simulink model "attitude_controller"  (R2015a)
settings: Solver=ode45  StartTime=0.0  StopTime=10.0  RelTol=1e-3
values from neighbouring files (symbols this model uses):
  AC_ATTITUDE_ACCEL_RP_CONTROLLER_MAX_RADSS = 720    [arducopter_initialization.m]    (also in startup.m)
  AC_ATTITUDE_ACCEL_RP_CONTROLLER_MIN_RADDS = 40    [arducopter_initialization.m]    (also in startup.m)
  AC_ATTITUDE_ACCEL_Y_CONTROLLER_MAX_RADSS = 120    [arducopter_initialization.m]    (also in startup.m)
  AC_ATTITUDE_ACCEL_Y_CONTROLLER_MIN_RADSS = 10    [arducopter_initialization.m]    (also in startup.m)
  ATC_ACCEL_P_MAX = 72000    [arducopter_initialization.m]    (also in startup.m)
  ATC_ACCEL_R_MAX = 72000    [arducopter_initialization.m]    (also in startup.m)
  ATC_ACCEL_Y_MAX = 36000    [arducopter_initialization.m]    (also in startup.m)
  ATC_ANG_PIT_P = 4.5000    (= 4.5)    [arducopter_initialization.m]    (also in startup.m)
  ATC_ANG_RLL_P = 4.5000    (= 4.5)    [arducopter_initialization.m]    (also in startup.m)
  ATC_ANG_YAW_P = 4.5000    (= 4.5)    [arducopter_initialization.m]    (also in startup.m)
  dt = 0.01    [arducopter_initialization.m]    (also in startup.m)
  p_angle_yaw_kp = 0.01    [arducopter_initialization.m]
  smoothing_gain = 1    [arducopter_initialization.m]    (also in startup.m)
undefined symbols (not defined in the file or in its folder): AC_ATTITUDE_THRUST_ERROR_ANGLE
libraries: arducopter_library x21, simulink x5, simulink_extras x4
settings Model: Creator=anne  LastModifiedBy=pa872d
settings DataIOCC: LimitDataPoints=off  SaveFormat=Dataset
settings HardwareCC: ProdBitPerPointer=64  ProdLargestAtomicFloat=Float  ProdIntDivRoundTo=Zero  ProdEndianess=LittleEndian  ProdHWDeviceType=Specified
settings ModelReferenceCC: PropagateSignalLabelsOutOfModel=on
settings GRTTargetCC: GeneratePreprocessorConditionals=Use local settings

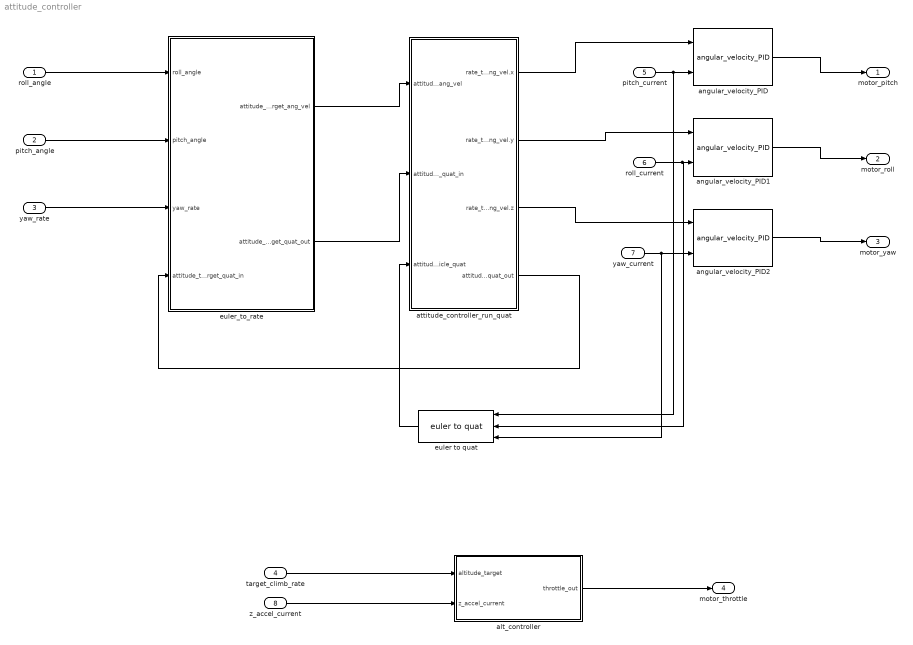
== system attitude_controller ==
  roll_angle : Inport
  pitch_angle : Inport  Port=2
  yaw_rate : Inport  Port=3
  target_climb_rate : Inport  Port=4
  pitch_current : Inport  Port=5
  roll_current : Inport  Port=6
  yaw_current : Inport  Port=7
  z_accel_current : Inport  Port=8
  alt_controller : Subsystem
  angular_velocity_PID : arducopter_library/angular_velocity_PID  P_rate=0  I_rate=0  D_rate=0  N=0
  angular_velocity_PID1 : arducopter_library/angular_velocity_PID  P_rate=0  I_rate=0  D_rate=0  N=0
  angular_velocity_PID2 : arducopter_library/angular_velocity_PID  P_rate=0  I_rate=0  D_rate=0  N=0
  attitude_controller_run_quat : Subsystem
  euler to quat : arducopter_library/euler to quat  SystemSampleTime=-1
  euler_to_rate : Subsystem  Variant=on
  motor_pitch : Outport
  motor_roll : Outport  Port=2
  motor_yaw : Outport  Port=3
  motor_throttle : Outport  Port=4
  wires:
  target_climb_rate/1 -> alt_controller/1(altitude_target)
  roll_angle/1 -> euler_to_rate/1(roll_angle)
  pitch_angle/1 -> euler_to_rate/2(pitch_angle)
  yaw_rate/1 -> euler_to_rate/3(yaw_rate)
  alt_controller/1(throttle_out) -> motor_throttle/1
  angular_velocity_PID2/1 -> motor_yaw/1
  angular_velocity_PID/1 -> motor_pitch/1
  angular_velocity_PID1/1 -> motor_roll/1
  yaw_current/1 -> euler to quat/3, angular_velocity_PID2/2
  pitch_current/1 -> euler to quat/1, angular_velocity_PID/2
  roll_current/1 -> euler to quat/2, angular_velocity_PID1/2
  z_accel_current/1 -> alt_controller/2(z_accel_current)
  attitude_controller_run_quat/1(rate_target_ang_vel.x) -> angular_velocity_PID/1
  attitude_controller_run_quat/2(rate_target_ang_vel.y) -> angular_velocity_PID1/1
  attitude_controller_run_quat/3(rate_target_ang_vel.z) -> angular_velocity_PID2/1
  attitude_controller_run_quat/4(attitude_target_quat_out) -> euler_to_rate/4(attitude_target_quat_in)
  euler_to_rate/2(attitude_target_quat_out) -> attitude_controller_run_quat/2(attitude_target_quat_in)
  euler_to_rate/1(attitude_target_ang_vel) -> attitude_controller_run_quat/1(attitude_target_ang_vel)
  euler to quat/1 -> attitude_controller_run_quat/3(attitude_vehicle_quat)

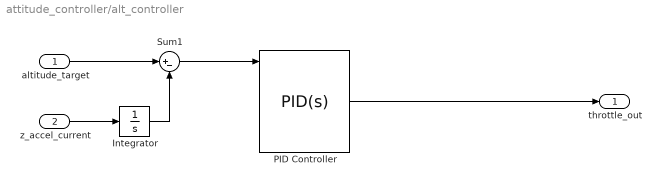
== system attitude_controller/alt_controller ==
  altitude_target : Inport
  z_accel_current : Inport  Port=2
  Integrator : Integrator
  PID Controller : simulink/Continuous/PID Controller  Controller=PID  TimeDomain=Continuous-time  SampleTime=-1  IntegratorMethod=Forward Euler  FilterMethod=Forward Euler  Form=Parallel  UseFilter=on  ControllerParametersSource=external  P=1  I=1  D=0  N=100  InitialConditionSource=internal  InitialConditionForIntegrator=0  InitialConditionForFilter=0  ExternalReset=none  LimitOutput=off  UpperSaturationLimit=inf  LowerSaturationLimit=-inf  LinearizeAsGain=on  AntiWindupMode=none  Kb=1  TrackingMode=off  Kt=1  PParamMin=[]  PParamMax=[]  IParamMin=[]  IParamMax=[]  DParamMin=[]  DParamMax=[]  NParamMin=[]  NParamMax=[]  KbParamMin=[]  KbParamMax=[]  KtParamMin=[]  KtParamMax=[]  POutMin=[]  POutMax=[]  IOutMin=[]  IOutMax=[]  DOutMin=[]  DOutMax=[]  NOutMin=[]  NOutMax=[]  KbOutMin=[]  KbOutMax=[]  KtOutMin=[]  KtOutMax=[]  IntegratorOutMin=[]  IntegratorOutMax=[]  FilterOutMin=[]  FilterOutMax=[]  SumOutMin=[]  SumOutMax=[]  SumI1OutMin=[]  SumI1OutMax=[]  SumI2OutMin=[]  SumI2OutMax=[]  SumI3OutMin=[]  SumI3OutMax=[]  SumDOutMin=[]  SumDOutMax=[]  SaturationOutMin=[]  SaturationOutMax=[]  IntegratorContinuousStateAttributes=''  IntegratorStateMustResolveToSignalObject=off  IntegratorRTWStateStorageClass=Auto  FilterContinuousStateAttributes=''  FilterStateMustResolveToSignalObject=off  FilterRTWStateStorageClass=Auto  DifferentiatorICPrevScaledInput=0  DifferentiatorOutMin=[]  DifferentiatorOutMax=[]
  Sum1 : Sum  Inputs=|+-
  throttle_out : Outport
  wires:
  PID Controller/1 -> throttle_out/1
  altitude_target/1 -> Sum1/1
  Sum1/1 -> PID Controller/1
  z_accel_current/1 -> Integrator/1
  Integrator/1 -> Sum1/2

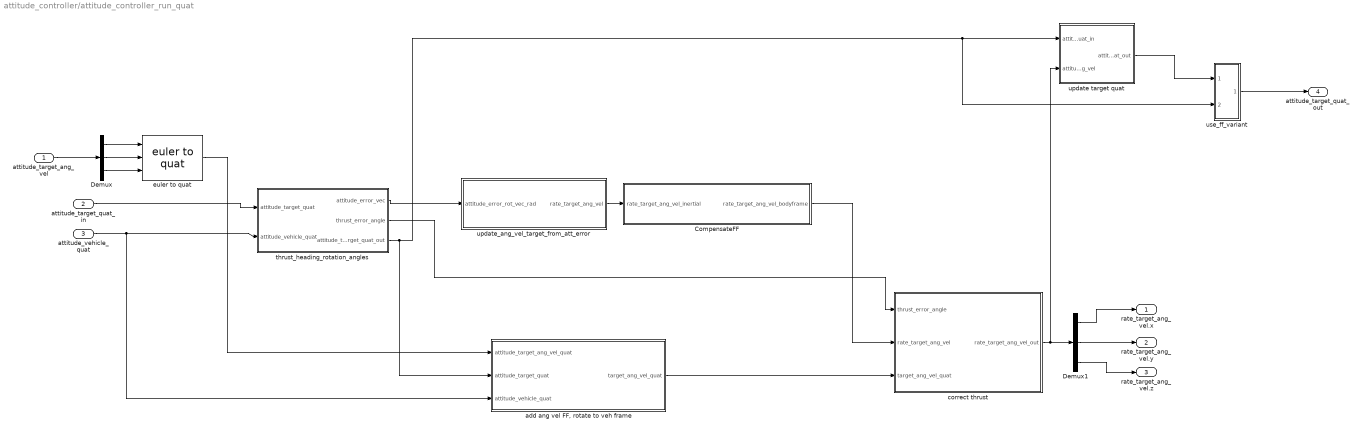
== system attitude_controller/attitude_controller_run_quat ==
  attitude_target_ang_vel : Inport
  attitude_target_quat_in : Inport  Port=2
  attitude_vehicle_quat : Inport  Port=3
  CompensateFF : Subsystem
  Demux : Demux  Outputs=3
  Demux1 : Demux  Outputs=3
  "add ang vel FF, rotate to veh frame" : MATLAB Function  TreatAsAtomicUnit=on
      settings: PermitHierarchicalResolution=ParametersOnly
  correct thrust : Subsystem
  euler to quat : arducopter_library/euler to quat  SystemSampleTime=-1
  thrust_heading_rotation_angles : Subsystem
  update target quat : Subsystem
  update_ang_vel_target_from_att_error : Subsystem  Variant=on
  use_ff_variant : Subsystem  Description=Replaced Block  mask(Replaced Block){}
      mask help: This block has been replaced with an empty subsystem because it used functionality that is unavailable in Simulink R2015a.
      mask Display: fprintf('Replaced: %s\n','VariantSource')
  rate_target_ang_vel.x : Outport
  rate_target_ang_vel.y : Outport  Port=2
  rate_target_ang_vel.z : Outport  Port=3
  attitude_target_quat_out : Outport  Port=4
  wires:
  attitude_target_ang_vel/1 -> Demux/1
  attitude_vehicle_quat/1 -> "add ang vel FF, rotate to veh frame"/3(attitude_vehicle_quat), thrust_heading_rotation_angles/2(attitude_vehicle_quat)
  attitude_target_quat_in/1 -> thrust_heading_rotation_angles/1(attitude_target_quat)
  thrust_heading_rotation_angles/1(attitude_error_vec) -> update_ang_vel_target_from_att_error/1(attitude_error_rot_vec_rad)
  Demux/1 -> euler to quat/1
  Demux/2 -> euler to quat/2
  Demux/3 -> euler to quat/3
  euler to quat/1 -> "add ang vel FF, rotate to veh frame"/1(attitude_target_ang_vel_quat)
  update_ang_vel_target_from_att_error/1(rate_target_ang_vel) -> CompensateFF/1(rate_target_ang_vel_inertial)
  "add ang vel FF, rotate to veh frame"/1(target_ang_vel_quat) -> correct thrust/3(target_ang_vel_quat)
  CompensateFF/1(rate_target_ang_vel_bodyframe) -> correct thrust/2(rate_target_ang_vel)
  thrust_heading_rotation_angles/2(thrust_error_angle) -> correct thrust/1(thrust_error_angle)
  correct thrust/1(rate_target_ang_vel_out) -> update target quat/2(attitude_target_ang_vel), Demux1/1
  Demux1/1 -> rate_target_ang_vel.x/1
  Demux1/2 -> rate_target_ang_vel.y/1
  Demux1/3 -> rate_target_ang_vel.z/1
  use_ff_variant/1(Out1) -> attitude_target_quat_out/1
  update target quat/1(attitude_target_quat_out) -> use_ff_variant/1(In1)
  thrust_heading_rotation_angles/3(attitude_target_quat_out) -> "add ang vel FF, rotate to veh frame"/2(attitude_target_quat), use_ff_variant/2(In2), update target quat/1(attitude_target_quat_in)

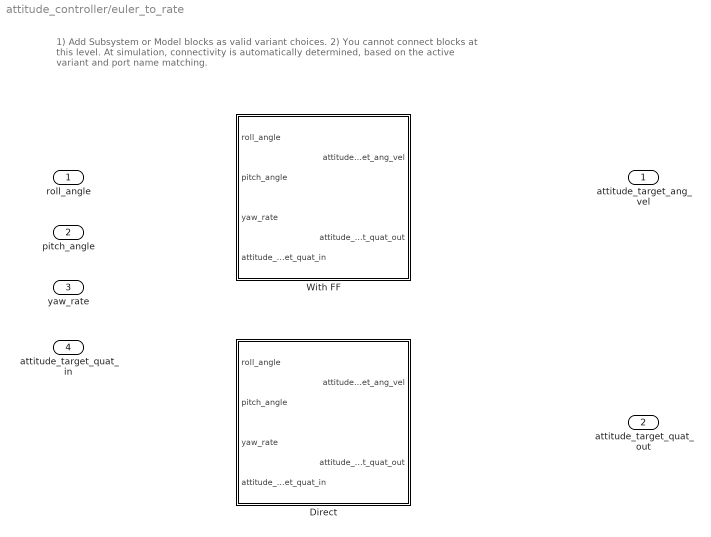
== system attitude_controller/euler_to_rate ==
  note: 1) Add Subsystem or Model blocks as valid variant choices.
      | 2) You cannot connect blocks at this level. At simulation, connectivity is automatically
      | determined, based on the active variant and port name matching.
  roll_angle : Inport
  pitch_angle : Inport  Port=2
  yaw_rate : Inport  Port=3
  attitude_target_quat_in : Inport  Port=4
  Direct : Subsystem  VariantControl=USE_DIRECT_VARIANT
  With FF : Subsystem  VariantControl=USE_FF_VARIANT
  attitude_target_ang_vel : Outport
  attitude_target_quat_out : Outport  Port=2

== system attitude_controller/attitude_controller_run_quat/CompensateFF ==
  note: This function should add a feed forward term that ensures the roll and pitch errors rotate with the body fram instead of the reference frame
  rate_target_ang_vel_inertial : Inport
  rate_target_ang_vel_bodyframe : Outport
  wires:
  rate_target_ang_vel_inertial/1 -> rate_target_ang_vel_bodyframe/1

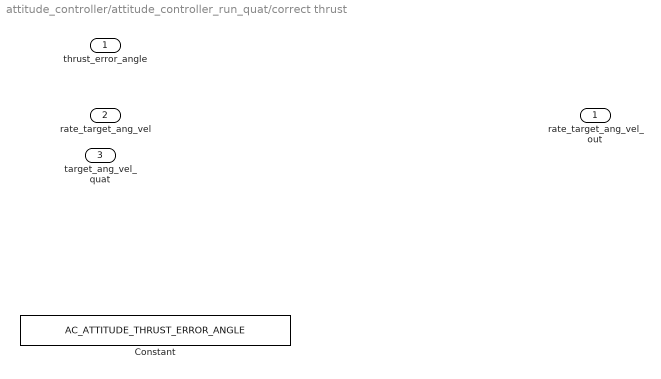
== system attitude_controller/attitude_controller_run_quat/correct thrust ==
  thrust_error_angle : Inport
  rate_target_ang_vel : Inport  Port=2
  target_ang_vel_quat : Inport  Port=3
  Constant : Constant  Value=AC_ATTITUDE_THRUST_ERROR_ANGLE
  rate_target_ang_vel_out : Outport

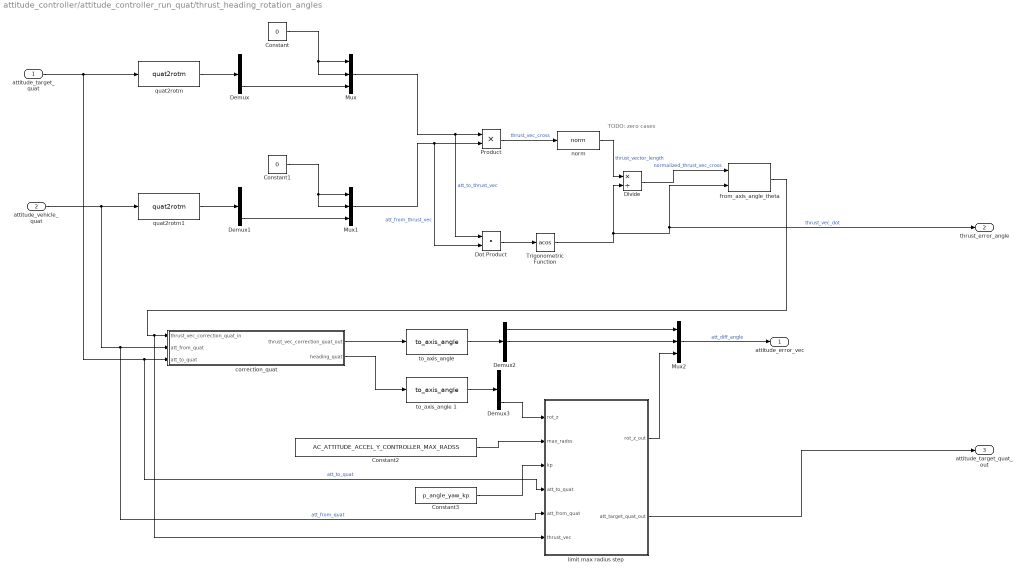
== system attitude_controller/attitude_controller_run_quat/thrust_heading_rotation_angles ==
  note: TODO: zero cases
  attitude_target_quat : Inport
  attitude_vehicle_quat : Inport  Port=2
  Constant : Constant  Value=0
  Constant1 : Constant  Value=0
  Constant2 : Constant  Value=AC_ATTITUDE_ACCEL_Y_CONTROLLER_MAX_RADSS
  Constant3 : Constant  Value=p_angle_yaw_kp
  Demux{,1..3} (4 alike) : Demux  Outputs=3
  Divide : Product  Inputs=*/
  Dot Product : DotProduct  OutMin=-1  OutMax=1  InputSameDT=on  OutDataTypeStr=Inherit: Inherit via internal rule
  Mux : Mux  Inputs=3
  Mux1 : Mux  Inputs=3
  Mux2 : Mux  Inputs=3
  Product : Product
  Trigonometric Function : Trigonometry  Operator=acos
  correction_quat : MATLAB Function  TreatAsAtomicUnit=on
      settings: PermitHierarchicalResolution=ParametersOnly
  from_axis_angle_theta : arducopter_library/from_axis_angle_theta
  limit max radius step : MATLAB Function  TreatAsAtomicUnit=on
      settings: PermitHierarchicalResolution=ParametersOnly
  "norm " : MATLABFcn  MATLABFcn=norm
  quat2rotm : arducopter_library/quat2rotm  SystemSampleTime=-1
  quat2rotm1 : arducopter_library/quat2rotm  SystemSampleTime=-1
  "to_axis_angle " : arducopter_library/to_axis_angle 
  to_axis_angle 1 : arducopter_library/to_axis_angle 
  attitude_error_vec : Outport
  thrust_error_angle : Outport  Port=2
  attitude_target_quat_out : Outport  Port=3
  wires:
  attitude_target_quat/1 -> limit max radius step/4(att_to_quat), correction_quat/3(att_to_quat), quat2rotm/1  "att_to_quat"
  attitude_vehicle_quat/1 -> limit max radius step/5(att_from_quat), correction_quat/2(att_from_quat), quat2rotm1/1  "att_from_quat"
  Mux2/1 -> attitude_error_vec/1  "att_diff_angle"
  Trigonometric Function/1 -> from_axis_angle_theta/2, thrust_error_angle/1, Divide/2  "thrust_vec_dot"
  quat2rotm/1 -> Demux/1
  Demux/3 -> Mux/3
  Constant/1 -> Mux/2, Mux/1
  Mux/1 -> Dot Product/1, Product/1  "att_to_thrust_vec"
  quat2rotm1/1 -> Demux1/1
  Demux1/3 -> Mux1/3
  Constant1/1 -> Mux1/2, Mux1/1
  Mux1/1 -> Dot Product/2, Product/2  "att_from_thrust_vec"
  Product/1 -> "norm "/1  "thrust_vec_cross"
  Dot Product/1 -> Trigonometric Function/1
  "norm "/1 -> Divide/1  "thrust_vector_length"
  Divide/1 -> from_axis_angle_theta/1  "normalized_thrust_vec_cross"
  from_axis_angle_theta/1 -> limit max radius step/6(thrust_vec), correction_quat/1(thrust_vec_correction_quat_in)
  correction_quat/1(thrust_vec_correction_quat_out) -> "to_axis_angle "/1
  "to_axis_angle "/1 -> Demux2/1
  Demux2/1 -> Mux2/1
  Demux2/2 -> Mux2/2
  correction_quat/2(heading_quat) -> to_axis_angle 1/1
  to_axis_angle 1/1 -> Demux3/1
  Demux3/3 -> limit max radius step/1(rot_z)
  Constant2/1 -> limit max radius step/2(max_radss)
  Constant3/1 -> limit max radius step/3(kp)
  limit max radius step/1(rot_z_out) -> Mux2/3
  limit max radius step/2(att_target_quat_out) -> attitude_target_quat_out/1

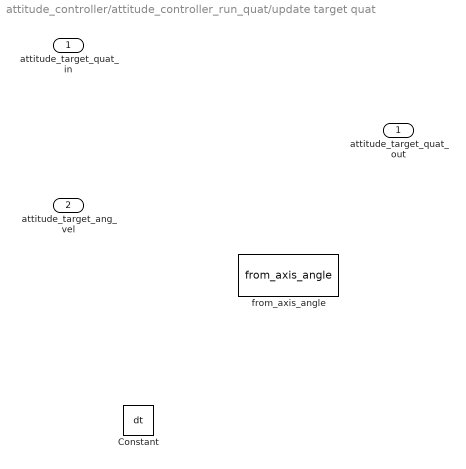
== system attitude_controller/attitude_controller_run_quat/update target quat ==
  attitude_target_quat_in : Inport
  attitude_target_ang_vel : Inport  Port=2
  Constant : Constant  Value=dt
  from_axis_angle : arducopter_library/from_axis_angle  SystemSampleTime=-1
  attitude_target_quat_out : Outport

== system attitude_controller/attitude_controller_run_quat/update_ang_vel_target_from_att_error ==
  note: 1) Add Subsystem or Model blocks as valid variant choices.
      | 2) You cannot connect blocks at this level. At simulation, connectivity is automatically
      | determined, based on the active variant and port name matching.
  attitude_error_rot_vec_rad : Inport
  shaped : Subsystem  VariantControl=USE_FF_VARIANT
  unshaped : Subsystem  VariantControl=USE_DIRECT_VARIANT
  rate_target_ang_vel : Outport

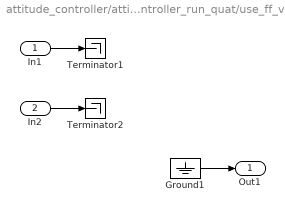
== system attitude_controller/attitude_controller_run_quat/use_ff_variant ==
  In1 : Inport
  In2 : Inport  Port=2
  Ground1 : Ground
  Terminator1 : Terminator
  Terminator2 : Terminator
  Out1 : Outport
  wires:
  Ground1/1 -> Out1/1
  In2/1 -> Terminator2/1
  In1/1 -> Terminator1/1

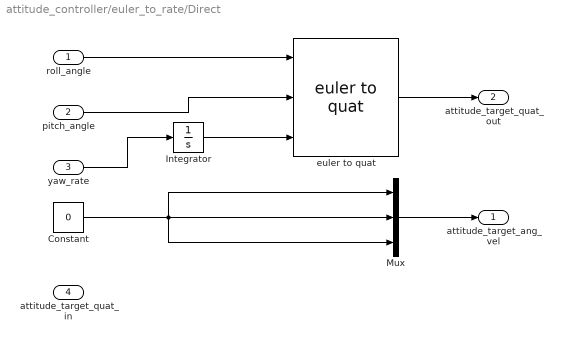
== system attitude_controller/euler_to_rate/Direct ==
  roll_angle : Inport
  pitch_angle : Inport  Port=2
  yaw_rate : Inport  Port=3
  attitude_target_quat_in : Inport  Port=4
  Constant : Constant  Value=0
  Integrator : Integrator
  Mux : Mux  Inputs=3
  euler to quat : arducopter_library/euler to quat  SystemSampleTime=-1
  attitude_target_ang_vel : Outport
  attitude_target_quat_out : Outport  Port=2
  wires:
  roll_angle/1 -> euler to quat/1
  pitch_angle/1 -> euler to quat/2
  Constant/1 -> Mux/3, Mux/2, Mux/1
  Integrator/1 -> euler to quat/3
  yaw_rate/1 -> Integrator/1
  euler to quat/1 -> attitude_target_quat_out/1
  Mux/1 -> attitude_target_ang_vel/1

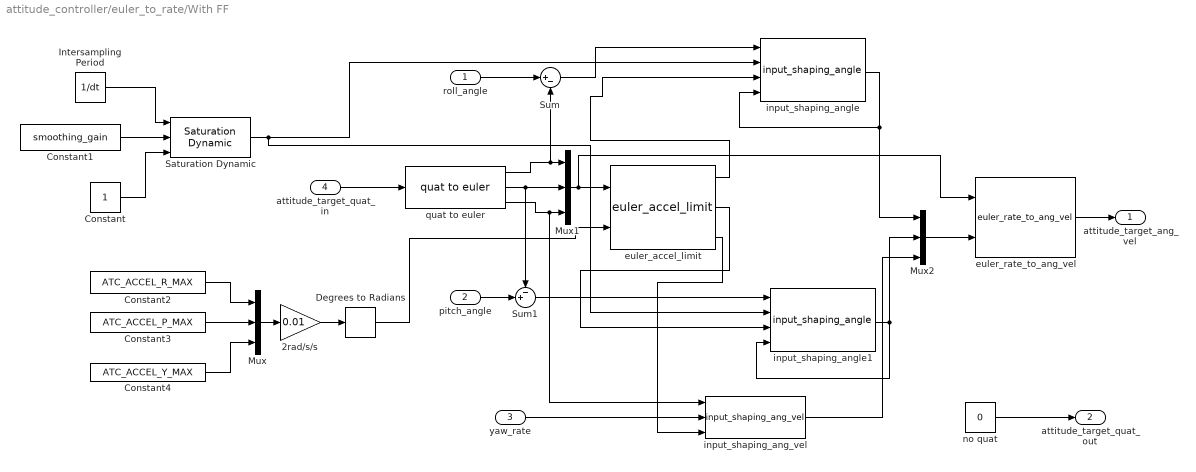
== system attitude_controller/euler_to_rate/With FF ==
  roll_angle : Inport
  pitch_angle : Inport  Port=2
  yaw_rate : Inport  Port=3
  attitude_target_quat_in : Inport  Port=4
  2rad/s/s : Gain  Gain=0.01
  Constant : Constant
  Constant1 : Constant  Value=smoothing_gain
  Constant2 : Constant  Value=ATC_ACCEL_R_MAX
  Constant3 : Constant  Value=ATC_ACCEL_P_MAX
  Constant4 : Constant  Value=ATC_ACCEL_Y_MAX
  Degrees to Radians : simulink_extras/Transformations/Degrees to Radians
  Intersampling Period : Constant  Value=1/dt
  Mux : Mux  Inputs=3
  Mux1 : Mux  Inputs=3
  Mux2 : Mux  Inputs=3
  Saturation Dynamic : simulink/Discontinuities/Saturation Dynamic  OutMin=[]  OutMax=[]  OutDataTypeStr=Inherit: Same as second input  OutDataType=fixdt(1, 16)  OutScaling=2^-10  DoSatur=off
  Sum : Sum  Inputs=|+-
  Sum1 : Sum  Inputs=-+|
  euler_accel_limit : arducopter_library/euler_accel_limit  SystemSampleTime=-1
  euler_rate_to_ang_vel : arducopter_library/euler_rate_to_ang_vel  SystemSampleTime=-1
  input_shaping_ang_vel : arducopter_library/input_shaping_ang_vel  SystemSampleTime=-1
  input_shaping_angle : arducopter_library/input_shaping_angle  SystemSampleTime=-1
  input_shaping_angle1 : arducopter_library/input_shaping_angle  SystemSampleTime=-1
  no quat : Constant  Value=0
  quat to euler : arducopter_library/quat to euler  SystemSampleTime=-1
  attitude_target_ang_vel : Outport
  attitude_target_quat_out : Outport  Port=2
  wires:
  Constant1/1 -> Saturation Dynamic/2
  attitude_target_quat_in/1 -> quat to euler/1
  Constant/1 -> Saturation Dynamic/3
  Intersampling Period/1 -> Saturation Dynamic/1
  roll_angle/1 -> Sum/1
  pitch_angle/1 -> Sum1/2
  yaw_rate/1 -> input_shaping_ang_vel/2
  quat to euler/1 -> Sum/2, Mux1/1
  quat to euler/2 -> Sum1/1, Mux1/2
  quat to euler/3 -> input_shaping_ang_vel/1, Mux1/3
  Mux1/1 -> euler_rate_to_ang_vel/1, euler_accel_limit/1
  Sum/1 -> input_shaping_angle/1
  Saturation Dynamic/1 -> input_shaping_angle1/2, input_shaping_angle/2
  euler_accel_limit/1 -> input_shaping_angle/3
  input_shaping_angle/1 -> Mux2/1, input_shaping_angle/4
  Sum1/1 -> input_shaping_angle1/1
  euler_accel_limit/2 -> input_shaping_angle1/3
  input_shaping_angle1/1 -> input_shaping_angle1/4, Mux2/2
  euler_accel_limit/3 -> input_shaping_ang_vel/3
  input_shaping_ang_vel/1 -> Mux2/3
  Mux2/1 -> euler_rate_to_ang_vel/2
  euler_rate_to_ang_vel/1 -> attitude_target_ang_vel/1
  no quat/1 -> attitude_target_quat_out/1
  Mux/1 -> 2rad/s/s/1
  Constant2/1 -> Mux/1
  Constant3/1 -> Mux/2
  Constant4/1 -> Mux/3
  2rad/s/s/1 -> Degrees to Radians/1
  Degrees to Radians/1 -> euler_accel_limit/2

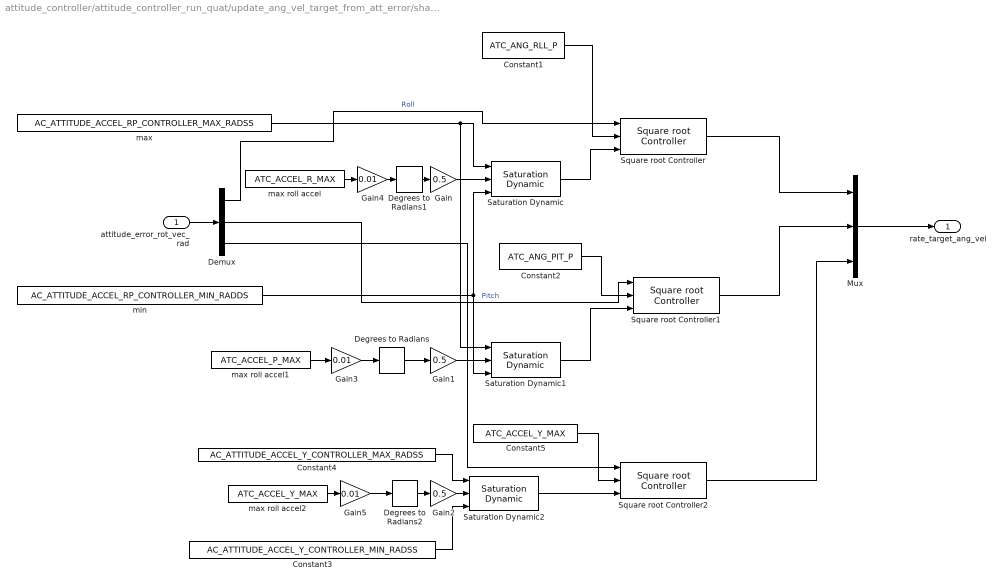
== system attitude_controller/attitude_controller_run_quat/update_ang_vel_target_from_att_error/shaped ==
  attitude_error_rot_vec_rad : Inport
  Constant1 : Constant  Value=ATC_ANG_RLL_P
  Constant2 : Constant  Value=ATC_ANG_PIT_P
  Constant3 : Constant  Value=AC_ATTITUDE_ACCEL_Y_CONTROLLER_MIN_RADSS
  Constant4 : Constant  Value=AC_ATTITUDE_ACCEL_Y_CONTROLLER_MAX_RADSS
  Constant5 : Constant  Value=ATC_ACCEL_Y_MAX
  Degrees to Radians : simulink_extras/Transformations/Degrees to Radians
  Degrees to Radians1 : simulink_extras/Transformations/Degrees to Radians
  Degrees to Radians2 : simulink_extras/Transformations/Degrees to Radians
  Demux : Demux  Outputs=3
  Gain : Gain  Gain=0.5
  Gain1 : Gain  Gain=0.5
  Gain2 : Gain  Gain=0.5
  Gain3 : Gain  Gain=0.01
  Gain4 : Gain  Gain=0.01
  Gain5 : Gain  Gain=0.01
  Mux : Mux  Inputs=3
  Saturation Dynamic : simulink/Discontinuities/Saturation Dynamic  OutMin=[]  OutMax=[]  OutDataTypeStr=Inherit: Same as second input  OutDataType=fixdt(1, 16)  OutScaling=2^-10  DoSatur=off
  Saturation Dynamic1 : simulink/Discontinuities/Saturation Dynamic  OutMin=[]  OutMax=[]  OutDataTypeStr=Inherit: Same as second input  OutDataType=fixdt(1, 16)  OutScaling=2^-10  DoSatur=off
  Saturation Dynamic2 : simulink/Discontinuities/Saturation Dynamic  OutMin=[]  OutMax=[]  OutDataTypeStr=Inherit: Same as second input  OutDataType=fixdt(1, 16)  OutScaling=2^-10  DoSatur=off
  Square root Controller : arducopter_library/Square root Controller  SystemSampleTime=-1
  Square root Controller1 : arducopter_library/Square root Controller  SystemSampleTime=-1
  Square root Controller2 : arducopter_library/Square root Controller  SystemSampleTime=-1
  max : Constant  Value=AC_ATTITUDE_ACCEL_RP_CONTROLLER_MAX_RADSS
  max roll accel : Constant  Value=ATC_ACCEL_R_MAX
  max roll accel1 : Constant  Value=ATC_ACCEL_P_MAX
  max roll accel2 : Constant  Value=ATC_ACCEL_Y_MAX
  min : Constant  Value=AC_ATTITUDE_ACCEL_RP_CONTROLLER_MIN_RADDS
  rate_target_ang_vel : Outport
  wires:
  attitude_error_rot_vec_rad/1 -> Demux/1
  Saturation Dynamic/1 -> Square root Controller/3
  Gain/1 -> Saturation Dynamic/2
  max/1 -> Saturation Dynamic1/1, Saturation Dynamic/1
  min/1 -> Saturation Dynamic/3, Saturation Dynamic1/3
  Demux/1 -> Square root Controller/1  "Roll"
  Saturation Dynamic1/1 -> Square root Controller1/3
  Gain1/1 -> Saturation Dynamic1/2
  Demux/2 -> Square root Controller1/1  "Pitch"
  Constant1/1 -> Square root Controller/2
  Constant2/1 -> Square root Controller1/2
  Saturation Dynamic2/1 -> Square root Controller2/3
  Gain2/1 -> Saturation Dynamic2/2
  Constant4/1 -> Saturation Dynamic2/1
  Constant3/1 -> Saturation Dynamic2/3
  Demux/3 -> Square root Controller2/1
  Constant5/1 -> Square root Controller2/2
  Mux/1 -> rate_target_ang_vel/1
  Square root Controller/1 -> Mux/1
  Square root Controller1/1 -> Mux/2
  Square root Controller2/1 -> Mux/3
  Gain3/1 -> Degrees to Radians/1
  max roll accel1/1 -> Gain3/1
  Degrees to Radians/1 -> Gain1/1
  Gain4/1 -> Degrees to Radians1/1
  max roll accel/1 -> Gain4/1
  Degrees to Radians1/1 -> Gain/1
  Gain5/1 -> Degrees to Radians2/1
  Degrees to Radians2/1 -> Gain2/1
  max roll accel2/1 -> Gain5/1

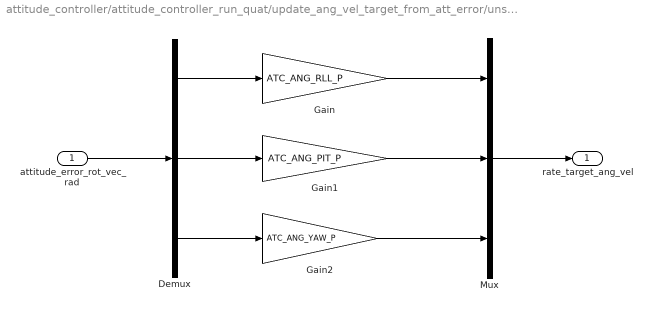
== system attitude_controller/attitude_controller_run_quat/update_ang_vel_target_from_att_error/unshaped ==
  attitude_error_rot_vec_rad : Inport
  Demux : Demux  Outputs=3
  Gain : Gain  Gain=ATC_ANG_RLL_P
  Gain1 : Gain  Gain=ATC_ANG_PIT_P
  Gain2 : Gain  Gain=ATC_ANG_YAW_P
  Mux : Mux  Inputs=3
  rate_target_ang_vel : Outport
  wires:
  attitude_error_rot_vec_rad/1 -> Demux/1
  Demux/1 -> Gain/1
  Gain/1 -> Mux/1
  Demux/2 -> Gain1/1
  Demux/3 -> Gain2/1
  Gain2/1 -> Mux/3
  Gain1/1 -> Mux/2
  Mux/1 -> rate_target_ang_vel/1

== matlab function attitude_controller/attitude_controller_run_quat/thrust_heading_rotation_angles/correction_quat ==
  data: thrust_vec_correction_quat_in input; thrust_vec_correction_quat_out output; att_from_quat input; heading_quat output; att_to_quat input
function [thrust_vec_correction_quat_out, heading_quat] = fcn(thrust_vec_correction_quat_in, att_from_quat, att_to_quat)
thrust_vec_correction_quat_out = att_from_quat \ thrust_vec_correction_quat_in * att_from_quat;

% calculate the remaining rotation required after thrust vector is rotated
heading_quat = thrust_vec_correction_quat_out \ att_from_quat \ att_to_quat;

== matlab function attitude_controller/attitude_controller_run_quat/add ang vel FF, rotate to veh frame ==
  data: attitude_target_ang_vel_quat input; attitude_target_quat input; target_ang_vel_quat output; attitude_vehicle_quat input
function target_ang_vel_quat = fcn(attitude_target_ang_vel_quat,...
                                attitude_target_quat, ...
                                attitude_vehicle_quat)


attitude_error_quat = inverse(attitude_vehicle_quat) * attitude_target_quat;
target_ang_vel_quat = inverse(attitude_error_quat) * ...
                        attitude_target_ang_vel_quat * attitude_error_quat;

== matlab function attitude_controller/attitude_controller_run_quat/thrust_heading_rotation_angles/limit max radius step ==
  data: rot_z input; rot_z_out output; max_radss input; kp input; att_to_quat input; att_from_quat input; thrust_vec input; att_target_quat_out output
function [rot_z_out, att_target_quat_out] = fcn(rot_z, max_radss, kp, att_to_quat, att_from_quat, thrust_vec)
red = max_radss/kp;
if abs(rot_z) > red;
    res = mod(rot_z, 2*pi);
    if res > pi
        res = res - 2*pi;
    end
    rot_z_out = max(min(rot_z,red, -red);
    
    % create rotation matrix for rotation about the vector v by angle theta
    vector = [0 0 rot_z_out];
    theta = norm(vector);
    if (theta == 0)
        heading_quat = [1 0 0 0];
    else
        vector = vector / theta;
        st2 = sin(theta/2);
        heading_quat = [cos(theta/2),
                vector(1) * st2,
                vector(2) * st2,
                vector(3) * st2];
    end
    att_target_quat_out = att_from_quat * thurst_vec * heading_quat;

else
    rot_z_out = rot_z;
    att_target_quat_out = att_to_quat;
end
